simulink model "sampleModel1453"  (R2023a)
settings: Solver=VariableStepAuto  StartTime=0.0  StopTime=10.0  RelTol=1e-3
libraries: simulink x6, hdlsllib x5
settings Model: Creator=user1  LastModifiedBy=user1

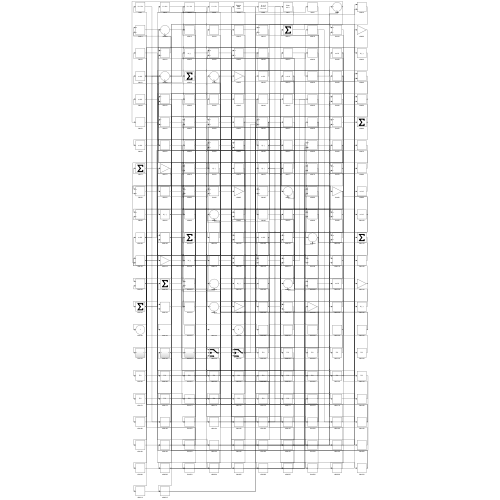
[thumbnail: Simulink's stored preview of the top-level diagram]
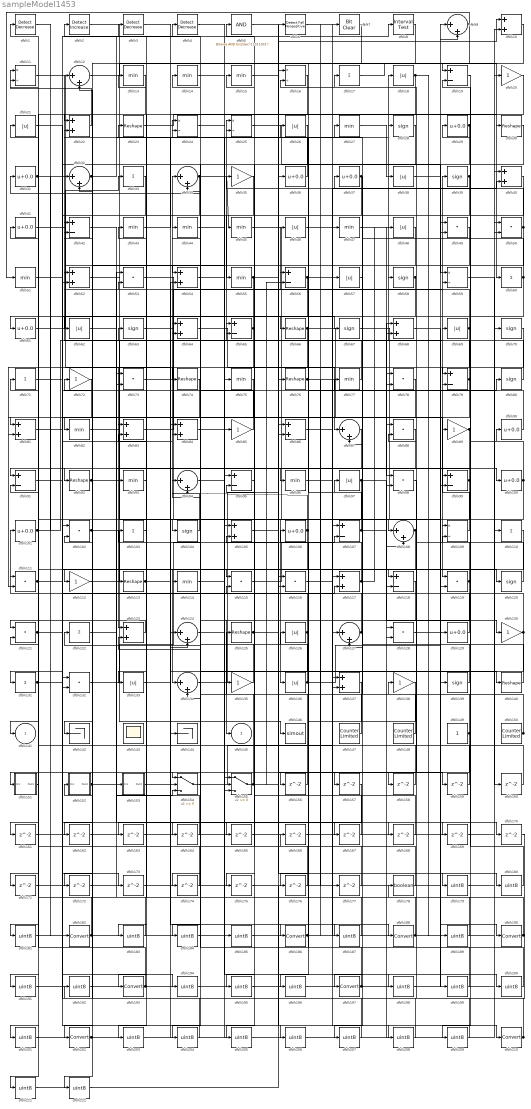
== system sampleModel1453 ==
  cfblk1 : simulink/Logic and Bit Operations/Detect Decrease  vinit=0.0  OutDataTypeStr=boolean
      settings: LibrarySourceBlock=|
      | hdlsllib/Logic and Bit
      | Operations/Detect
      | Decrease
  cfblk{10,22,40,52,54,64,68,81,83..84,86,105,117,123,137} (15 alike) : Sum
  cfblk{29,31,36..37,41,61,90,100..101,106,129} (11 alike) : Bias  Bias=0.0  SaturateOnIntegerOverflow=off
  cfblk{49..50,53,73,78,88,98,102,111,115..116,119,121,128,132} (15 alike) : DotProduct  OutDataTypeStr=Inherit: Inherit via internal rule
  cfblk{17,33,60,71,103,110,122,131} (8 alike) : Sum  Inputs=+
  cfblk{28,39,58,63,67,70,80,104,120,139} (10 alike) : Signum
  cfblk{19,42,56,65,79,91,95,99,107,118} (10 alike) : Sum  Inputs=+-
  cfblk{9,12,32,34,87,94,108,124,127,134} (10 alike) : Sum  Inputs=|++
  cfblk{11,16,24..25,59,109} (6 alike) : Product  Inputs=*/  RndMeth=Zero  SaturateOnIntegerOverflow=on
  cfblk{20,35,72,85,89,112,130,135,138} (9 alike) : Gain
  cfblk{23,30,66,74,76,92,113,125,140} (9 alike) : Reshape
  cfblk{13..15,27,43..45,47,51,55,75,77,82,93,96,114} (16 alike) : MinMax
  cfblk{18,21,26,38,46,48,57,62,69,97,126,133,136} (13 alike) : Abs  SaturateOnIntegerOverflow=off
  cfblk142 : Terminator
  cfblk143 : Scope
      settings: Floating=on
  cfblk144 : Terminator
  cfblk146 : ToWorkspace  VariableName=simout  SaveFormat=Timeseries  SampleTime=-1
  cfblk147 : hdlsllib/Sources/Counter Limited  uplimit=7  tsamp=-1
  cfblk148 : hdlsllib/Sources/Counter Limited  uplimit=7  tsamp=-1
  cfblk149 : Constant  SampleTime=-1
  cfblk150 : hdlsllib/Sources/Counter Limited  uplimit=7  tsamp=-1
  cfblk151 : Subsystem
      settings: LibrarySourceBlock=|
      | hdlsllib/Ports &
      | Subsystems/Subsystem
  cfblk152 : Subsystem
      settings: LibrarySourceBlock=|
      | hdlsllib/Ports &
      | Subsystems/Subsystem
  cfblk153 : Subsystem
      settings: LibrarySourceBlock=|
      | hdlsllib/Ports &
      | Subsystems/Subsystem
  cfblk154 : Switch  SaturateOnIntegerOverflow=off  InputSameDT=off
  cfblk155 : Switch  SaturateOnIntegerOverflow=off  InputSameDT=off
  cfblk{156..177} (22 alike) : Delay  SampleTime=1
  cfblk178 : DataTypeConversion  OutDataTypeStr=boolean  SaturateOnIntegerOverflow=off  RndMeth=Floor
  cfblk{179..181,183..185,187,189,191..192,194..196,198..201,203..209,211..212} (26 alike) : DataTypeConversion  OutDataTypeStr=uint8  SaturateOnIntegerOverflow=off  RndMeth=Floor
  cfblk{182,186,188,190,193,197,202,210} (8 alike) : DataTypeConversion  SaturateOnIntegerOverflow=off  RndMeth=Floor
  cfblk2 : simulink/Logic and Bit Operations/Detect Increase  vinit=0.0  OutDataTypeStr=boolean
      settings: LibrarySourceBlock=|
      | hdlsllib/Logic and Bit
      | Operations/Detect
      | Increase
  cfblk3 : simulink/Logic and Bit Operations/Detect Decrease  vinit=0.0  OutDataTypeStr=boolean
      settings: LibrarySourceBlock=|
      | hdlsllib/Logic and Bit
      | Operations/Detect
      | Decrease
  cfblk4 : simulink/Logic and Bit Operations/Detect Decrease  vinit=0.0  OutDataTypeStr=boolean
      settings: LibrarySourceBlock=|
      | hdlsllib/Logic and Bit
      | Operations/Detect
      | Decrease
  cfblk5 : simulink/Logic and Bit Operations/Bitwise Operator  logicop=AND  UseBitMask=on  BitMask=bin2dec('11011001')  BitMaskRealWorld=Stored Integer
      settings: LibrarySourceBlock=|
      | hdlsllib/Logic and Bit
      | Operations/Bitwise
      | Operator
  cfblk6 : hdlsllib/Logic and Bit Operations/Detect Fall Nonpositive  vinit=0  OutDataTypeStr=boolean
  cfblk7 : simulink/Logic and Bit Operations/Bit Clear  iBit=0
      settings: LibrarySourceBlock=|
      | hdlsllib/Logic and Bit
      | Operations/Bit Clear
  cfblk8 : hdlsllib/Logic and Bit Operations/Interval Test  IntervalClosedRight=on  uplimit=0.5  IntervalClosedLeft=on  lowlimit=-0.5  OutDataTypeStr=boolean
  cfblk141 : Outport  VectorParamsAs1DForOutWhenUnconnected=off
  cfblk145 : Outport  Port=2  VectorParamsAs1DForOutWhenUnconnected=off
  wires:
  cfblk102/1 -> cfblk146/1, cfblk118/1
  cfblk109/1 -> cfblk39/1
  cfblk22/1 -> cfblk11/1
  cfblk2/1 -> cfblk104/1
  cfblk155/1 -> cfblk36/1, cfblk31/1, cfblk56/2
  cfblk61/1 -> cfblk33/1
  cfblk25/1 -> cfblk59/1
  cfblk100/1 -> cfblk90/1, cfblk79/2, cfblk118/2, cfblk191/1
  cfblk9/1 -> cfblk51/1, cfblk155/3
  cfblk65/1 -> cfblk61/1, cfblk73/2, cfblk64/2
  cfblk101/1 -> cfblk63/1, cfblk32/1
  cfblk108/1 -> cfblk134/1, cfblk201/1
  cfblk41/1 -> cfblk123/1
  cfblk92/1 -> cfblk18/1, cfblk170/1
  cfblk103/1 -> cfblk23/1
  cfblk97/1 -> cfblk136/1, cfblk108/2
  cfblk72/1 -> cfblk131/1
  cfblk132/1 -> cfblk16/1
  cfblk112/1 -> cfblk25/1
  cfblk17/1 -> cfblk60/1
  cfblk74/1 -> cfblk81/1
  cfblk64/1 -> cfblk87/1
  cfblk12/1 -> cfblk19/1
  cfblk53/1 -> cfblk127/1
  cfblk104/1 -> cfblk34/1
  cfblk119/1 -> cfblk17/1, cfblk174/1
  cfblk105/1 -> cfblk59/2
  cfblk66/1 -> cfblk119/1, cfblk40/2, cfblk175/1
  cfblk89/1 -> cfblk91/1, cfblk181/1
  cfblk117/1 -> cfblk15/1, cfblk48/1
  cfblk48/1 -> cfblk112/1
  cfblk35/1 -> cfblk55/1
  cfblk136/1 -> cfblk9/1, cfblk2/1
  cfblk1/1 -> cfblk182/1
  cfblk115/1 -> cfblk107/2
  cfblk52/1 -> cfblk137/1
  cfblk55/1 -> cfblk114/1, cfblk159/1
  cfblk23/1 -> cfblk30/1
  cfblk71/1 -> cfblk89/1
  cfblk36/1 -> cfblk13/1
  cfblk90/1 -> cfblk26/1
  cfblk118/1 -> cfblk145/1
  cfblk116/1 -> cfblk210/1
  cfblk111/1 -> cfblk84/2, cfblk165/1
  cfblk99/1 -> cfblk93/1, cfblk176/1
  cfblk38/1 -> cfblk9/2
  cfblk150/1 -> cfblk97/1, cfblk123/2
  cfblk58/1 -> cfblk127/2, cfblk53/2
  cfblk30/1 -> cfblk54/1
  cfblk16/1 -> cfblk141/1
  cfblk154/1 -> cfblk57/1
  cfblk76/1 -> cfblk129/1, cfblk177/1
  cfblk40/1 -> cfblk113/1
  cfblk45/1 -> cfblk137/2
  cfblk19/1 -> cfblk109/1
  cfblk125/1 -> cfblk86/1, cfblk58/1
  cfblk18/1 -> cfblk32/2, cfblk189/1
  cfblk7/1 -> cfblk92/1
  cfblk15/1 -> cfblk10/1
  cfblk3/1 -> cfblk186/1
  cfblk82/1 -> cfblk144/1
  cfblk34/1 -> cfblk45/1, cfblk172/1
  cfblk11/1 -> cfblk124/1
  cfblk80/1 -> cfblk44/1
  cfblk44/1 -> cfblk108/1
  cfblk113/1 -> cfblk140/1, cfblk168/1
  cfblk67/1 -> cfblk139/1
  cfblk130/1 -> cfblk111/1, cfblk164/1
  cfblk151/1(Out1) -> cfblk21/1
  cfblk134/1 -> cfblk76/1
  cfblk95/1 -> cfblk65/1
  cfblk32/1 -> cfblk4/1, cfblk24/2
  cfblk149/1 -> cfblk125/1, cfblk211/1
  cfblk85/1 -> cfblk34/2
  cfblk94/1 -> cfblk105/1
  cfblk148/1 -> cfblk126/1
  cfblk49/1 -> cfblk154/1
  cfblk8/1 -> cfblk96/1
  cfblk60/1 -> cfblk27/1, cfblk74/1
  cfblk56/1 -> cfblk120/1, cfblk162/1, cfblk163/1
  cfblk75/1 -> cfblk202/1
  cfblk79/1 -> cfblk81/2, cfblk42/2
  cfblk28/1 -> cfblk83/1
  cfblk127/1 -> cfblk43/1, cfblk42/1
  cfblk20/1 -> cfblk193/1
  cfblk42/1 -> cfblk153/1(In1)
  cfblk147/1 -> cfblk122/1
  cfblk54/1 -> cfblk66/1
  cfblk73/1 -> cfblk46/1
  cfblk126/1 -> cfblk101/1, cfblk135/1
  cfblk69/1 -> cfblk12/1, cfblk142/1, cfblk111/2
  cfblk124/1 -> cfblk28/1
  cfblk86/1 -> cfblk99/1
  cfblk14/1 -> cfblk188/1
  cfblk77/1 -> cfblk52/1
  cfblk135/1 -> cfblk103/1
  cfblk63/1 -> cfblk86/2
  cfblk131/1 -> cfblk77/1, cfblk8/1
  cfblk83/1 -> cfblk69/1
  cfblk33/1 -> cfblk82/1
  cfblk50/1 -> cfblk35/1, cfblk62/1
  cfblk91/1 -> cfblk115/1
  cfblk133/1 -> cfblk154/2
  cfblk47/1 -> cfblk98/1
  cfblk120/1 -> cfblk16/2
  cfblk138/1 -> cfblk197/1
  cfblk123/1 -> cfblk121/1
  cfblk62/1 -> cfblk100/1
  cfblk29/1 -> cfblk132/2, cfblk79/1
  cfblk129/1 -> cfblk37/1
  cfblk31/1 -> cfblk85/1, cfblk173/1
  cfblk10/1 -> cfblk22/1
  cfblk140/1 -> cfblk24/1
  cfblk106/1 -> cfblk94/2, cfblk151/1(In1), cfblk161/1
  cfblk87/1 -> cfblk133/1
  cfblk46/1 -> cfblk99/2
  cfblk122/1 -> cfblk80/1
  cfblk39/1 -> cfblk156/1, cfblk209/1
  cfblk128/1 -> cfblk190/1
  cfblk152/1(Out1) -> cfblk154/3, cfblk212/1
  cfblk43/1 -> cfblk25/2
  cfblk21/1 -> cfblk67/1
  cfblk81/1 -> cfblk64/1
  cfblk27/1 -> cfblk38/1
  cfblk37/1 -> cfblk52/2, cfblk87/2
  cfblk121/1 -> cfblk117/2, cfblk206/1
  cfblk139/1 -> cfblk105/2
  cfblk107/1 -> cfblk56/1, cfblk130/1
  cfblk156/1 -> cfblk22/2
  cfblk57/1 -> cfblk157/1
  cfblk98/1 -> cfblk158/1
  cfblk158/1 -> cfblk65/2
  cfblk159/1 -> cfblk121/2
  cfblk59/1 -> cfblk160/1
  cfblk160/1 -> cfblk109/2
  cfblk161/1 -> cfblk50/2
  cfblk162/1 -> cfblk117/1
  cfblk163/1 -> cfblk124/2
  cfblk164/1 -> cfblk73/1
  cfblk165/1 -> cfblk95/2
  cfblk166/1 -> cfblk10/2
  cfblk24/1 -> cfblk167/1
  cfblk167/1 -> cfblk107/1
  cfblk168/1 -> cfblk115/2
  cfblk153/1(Out1) -> cfblk169/1
  cfblk169/1 -> cfblk19/2
  cfblk13/1 -> cfblk171/1
  cfblk171/1 -> cfblk119/2
  cfblk172/1 -> cfblk155/1
  cfblk173/1 -> cfblk155/2
  cfblk174/1 -> cfblk11/2
  cfblk176/1 -> cfblk83/2
  cfblk177/1 -> cfblk134/2
  cfblk178/1 -> cfblk5/1
  cfblk5/1 -> cfblk179/1
  cfblk179/1 -> cfblk40/1
  cfblk6/1 -> cfblk180/1
  cfblk180/1 -> cfblk29/1
  cfblk181/1 -> cfblk6/1
  cfblk182/1 -> cfblk12/2, cfblk41/1
  cfblk157/1 -> cfblk183/1
  cfblk183/1 -> cfblk1/1
  cfblk70/1 -> cfblk184/1
  cfblk184/1 -> cfblk47/1
  cfblk114/1 -> cfblk185/1
  cfblk185/1 -> cfblk70/1
  cfblk186/1 -> cfblk166/1, cfblk98/2, cfblk7/1
  cfblk84/1 -> cfblk187/1
  cfblk187/1 -> cfblk3/1
  cfblk188/1 -> cfblk178/1, cfblk102/2, cfblk53/1
  cfblk189/1 -> cfblk14/1
  cfblk190/1 -> cfblk84/1, cfblk91/2
  cfblk191/1 -> cfblk128/1
  cfblk170/1 -> cfblk192/1
  cfblk192/1 -> cfblk128/2
  cfblk193/1 -> cfblk71/1, cfblk132/1
  cfblk51/1 -> cfblk194/1
  cfblk194/1 -> cfblk20/1
  cfblk110/1 -> cfblk195/1
  cfblk195/1 -> cfblk49/1
  cfblk137/1 -> cfblk196/1
  cfblk196/1 -> cfblk110/1
  cfblk197/1 -> cfblk49/2, cfblk94/1
  cfblk4/1 -> cfblk198/1
  cfblk198/1 -> cfblk138/1
  cfblk68/1 -> cfblk199/1
  cfblk199/1 -> cfblk106/1
  cfblk96/1 -> cfblk200/1
  cfblk200/1 -> cfblk68/1
  cfblk201/1 -> cfblk68/2
  cfblk202/1 -> cfblk54/2, cfblk50/1
  cfblk93/1 -> cfblk203/1
  cfblk203/1 -> cfblk75/1
  cfblk78/1 -> cfblk204/1
  cfblk204/1 -> cfblk72/1
  cfblk26/1 -> cfblk205/1
  cfblk205/1 -> cfblk78/1
  cfblk206/1 -> cfblk78/2
  cfblk88/1 -> cfblk207/1
  cfblk207/1 -> cfblk152/1(In1)
  cfblk175/1 -> cfblk208/1
  cfblk208/1 -> cfblk88/1
  cfblk209/1 -> cfblk88/2
  cfblk210/1 -> cfblk102/1, cfblk95/1
  cfblk211/1 -> cfblk116/1
  cfblk212/1 -> cfblk116/2

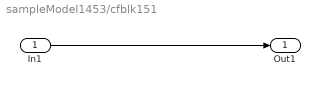
== system sampleModel1453/cfblk151 ==
  In1 : Inport
  Out1 : Outport
  wires:
  In1/1 -> Out1/1

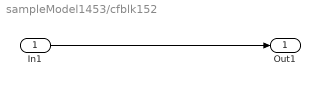
== system sampleModel1453/cfblk152 ==
  In1 : Inport
  Out1 : Outport
  wires:
  In1/1 -> Out1/1

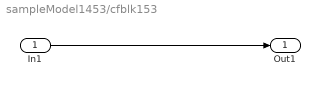
== system sampleModel1453/cfblk153 ==
  In1 : Inport
  Out1 : Outport
  wires:
  In1/1 -> Out1/1
